simulink model "rocket_engine_simulation"  (R2024b)
settings: Solver=ode45  StartTime=0.0  StopTime=sim_time  RelTol=1e-3
values from neighbouring files (symbols this model uses):
  initial_propellant_mass = 1000    [rocket_parameters.m]
  P_c = 7e6    (= 7000000)    [rocket_parameters.m]
  rocket_dry_mass = 500    [rocket_parameters.m]
  T_c = 3500    [rocket_parameters.m]
settings Model: Creator=Venika  LastModifiedBy=Venika

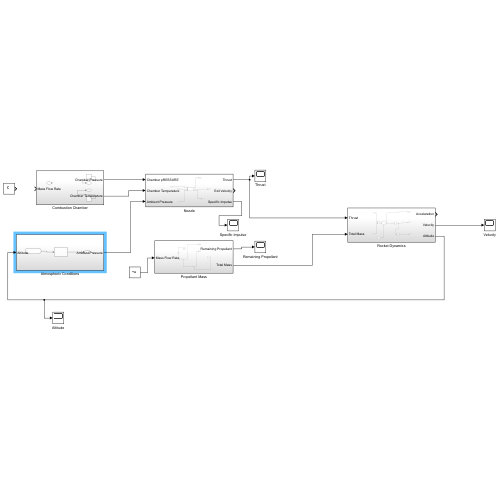
[thumbnail: Simulink's stored preview of the top-level diagram]
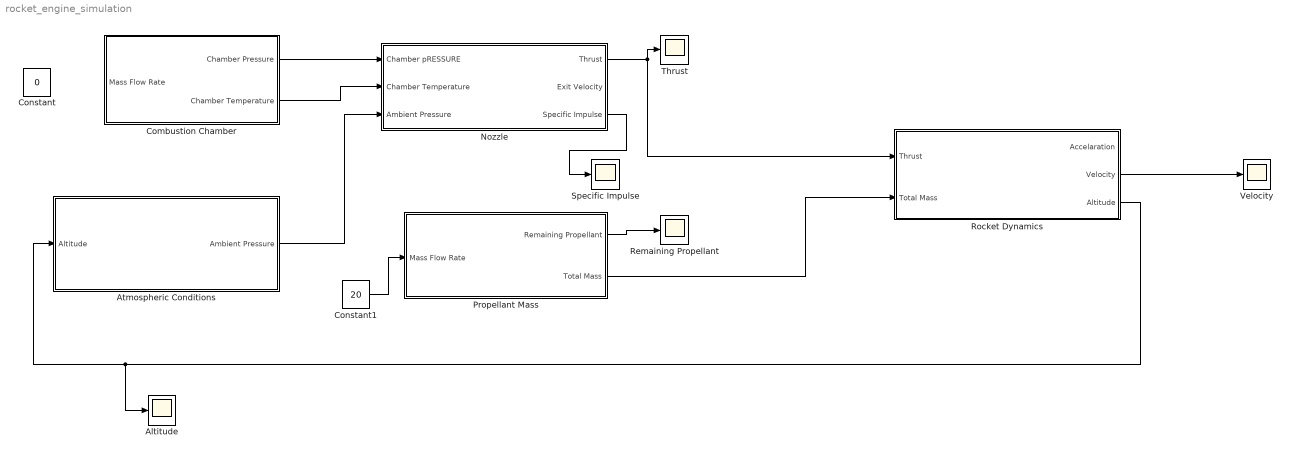
== system rocket_engine_simulation ==
  Altitude : Scope
  Atmospheric Conditions : Subsystem
  Combustion Chamber : Subsystem
  Constant : Constant  Value=0
  Constant1 : Constant  Value=20
  Nozzle : Subsystem
  Propellant Mass : Subsystem
  Remaining Propellant : Scope
  Rocket Dynamics : Subsystem
  Specific Impulse : Scope
  Thrust : Scope
  Velocity : Scope
  wires:
  Combustion Chamber/1(Chamber Pressure) -> Nozzle/1("Chamber pRESSURE ")
  Combustion Chamber/2(Chamber Temperature) -> Nozzle/2(Chamber Temperature)
  Rocket Dynamics/3(Altitude) -> Altitude/1, Atmospheric Conditions/1(Altitude)
  Atmospheric Conditions/1(Ambient Pressure) -> Nozzle/3(Ambient Pressure)
  Constant1/1 -> Propellant Mass/1(Mass Flow Rate)
  Nozzle/1(Thrust) -> Rocket Dynamics/1(Thrust), Thrust/1
  Propellant Mass/2(Total Mass) -> Rocket Dynamics/2(Total Mass)
  Nozzle/3(Specific Impulse) -> Specific Impulse/1
  Propellant Mass/1(Remaining Propellant) -> Remaining Propellant/1
  Rocket Dynamics/2(Velocity) -> Velocity/1

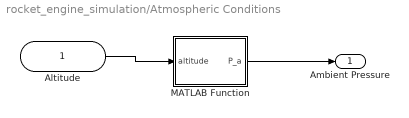
== system rocket_engine_simulation/Atmospheric Conditions ==
  Altitude : Inport
  MATLAB Function : MATLAB Function  TreatAsAtomicUnit=on
  Ambient Pressure : Outport
  wires:
  Altitude/1 -> MATLAB Function/1(altitude)
  MATLAB Function/1(P_a) -> Ambient Pressure/1

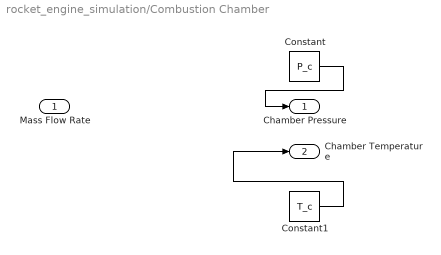
== system rocket_engine_simulation/Combustion Chamber ==
  Mass Flow Rate : Inport
  Constant : Constant  Value=P_c
  Constant1 : Constant  Value=T_c
  Chamber Pressure : Outport
  Chamber Temperature : Outport  Port=2
  wires:
  Constant/1 -> Chamber Pressure/1
  Constant1/1 -> Chamber Temperature/1

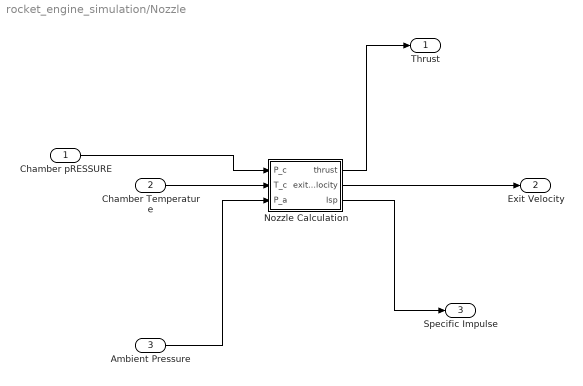
== system rocket_engine_simulation/Nozzle ==
  "Chamber pRESSURE " : Inport
  Chamber Temperature : Inport  Port=2
  Ambient Pressure : Inport  Port=3
  Nozzle Calculation : MATLAB Function  TreatAsAtomicUnit=on
  Thrust : Outport
  Exit Velocity : Outport  Port=2
  Specific Impulse : Outport  Port=3
  wires:
  "Chamber pRESSURE "/1 -> Nozzle Calculation/1(P_c)
  Chamber Temperature/1 -> Nozzle Calculation/2(T_c)
  Ambient Pressure/1 -> Nozzle Calculation/3(P_a)
  Nozzle Calculation/1(thrust) -> Thrust/1
  Nozzle Calculation/2(exit_velocity) -> Exit Velocity/1
  Nozzle Calculation/3(Isp) -> Specific Impulse/1

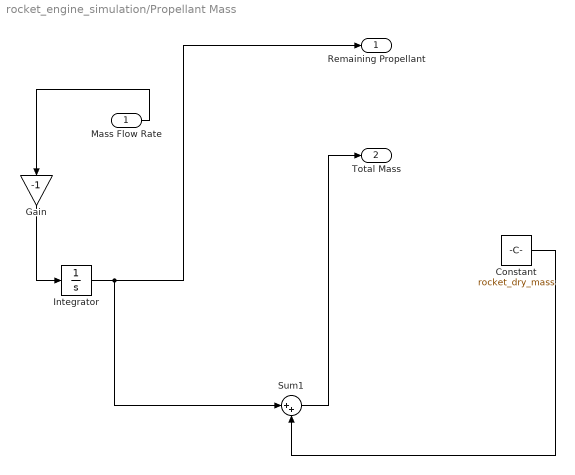
== system rocket_engine_simulation/Propellant Mass ==
  Mass Flow Rate : Inport
  Constant : Constant  Value=rocket_dry_mass
  Gain : Gain  Gain=-1
  Integrator : Integrator  InitialCondition=initial_propellant_mass
  Sum1 : Sum  Inputs=|++
  Remaining Propellant : Outport
  Total Mass : Outport  Port=2
  wires:
  Mass Flow Rate/1 -> Gain/1
  Gain/1 -> Integrator/1
  Integrator/1 -> Sum1/1, Remaining Propellant/1
  Constant/1 -> Sum1/2
  Sum1/1 -> Total Mass/1

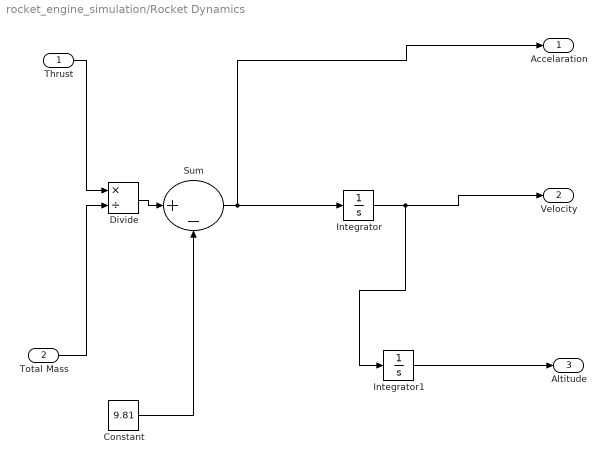
== system rocket_engine_simulation/Rocket Dynamics ==
  Thrust : Inport
  Total Mass : Inport  Port=2
  Constant : Constant  Value=9.81
  Divide : Product  Inputs=*/
  Integrator : Integrator
  Integrator1 : Integrator
  Sum : Sum  Inputs=|+-
  Accelaration : Outport
  Velocity : Outport  Port=2
  Altitude : Outport  Port=3
  wires:
  Thrust/1 -> Divide/1
  Total Mass/1 -> Divide/2
  Divide/1 -> Sum/1
  Constant/1 -> Sum/2
  Sum/1 -> Accelaration/1, Integrator/1
  Integrator/1 -> Integrator1/1, Velocity/1
  Integrator1/1 -> Altitude/1

== matlab function rocket_engine_simulation/Atmospheric Conditions/MATLAB Function ==
  data: altitude input; P_a output
function P_a = fcn(altitude)
    % Standard atmospheric model (simplified)
    if altitude <= 11000
        % Troposphere
        T = 288.15 - 0.0065 * altitude;
        P_a = 101325 * (T/288.15)^5.2561;
    else
        % Simplified upper atmosphere
        P_a = 22632 * exp(-0.0001577 * (altitude - 11000));
    end
end

== matlab function rocket_engine_simulation/Nozzle/Nozzle Calculation ==
  data: P_c input; thrust output; T_c input; P_a input; exit_velocity output; Isp output
function [thrust, exit_velocity, Isp] = fcn(P_c, T_c, P_a)
    % Constants
    gamma = 1.2;         % Specific heat ratio
    R = 287;             % Gas constant (J/kg·K)
    g0 = 9.81;           % Standard gravity (m/s²)
    A_t = 0.01;          % Throat area (m²)
    epsilon = 15;        % Nozzle expansion ratio
    A_e = A_t * epsilon; % Exit area (m²)
    m_dot = 20;          % Mass flow rate (kg/s)
    
    % Calculate pressure ratio for optimal expansion
    P_e_P_c_opt = (1 + (gamma-1)/2)^(-gamma/(gamma-1));
    
    % Calculate actual exit pressure (assuming isentropic flow)
    P_e = P_c * (1 + (gamma-1)/2 * (1/epsilon)^((gamma-1)/gamma))^(-gamma/(gamma-1));
    
    % Calculate exit velocity
    exit_velocity = sqrt(2*gamma*R*T_c/(gamma-1)*(1-(P_e/P_c)^((gamma-1)/gamma)));
    
    % Calculate thrust
    thrust = m_dot * exit_velocity + (P_e - P_a) * A_e;
    
    % Calculate specific impulse
    Isp = thrust / (m_dot * g0);
end
